simulink model "BSP_v2"  (R2024b)
settings: Solver=VariableStepAuto  StartTime=0.0  StopTime=10.0  RelTol=1e-3
settings Model: Creator=satyendra  LastModifiedBy=satyendra

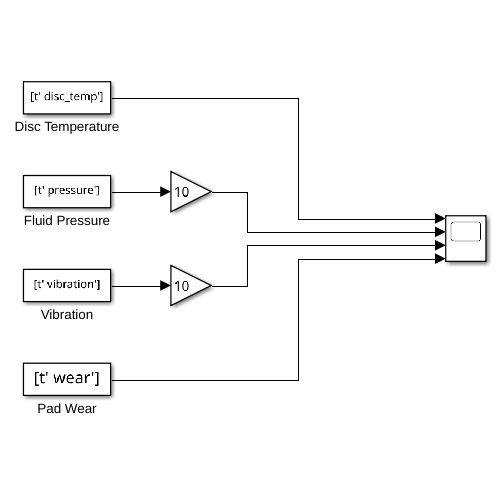
[thumbnail: Simulink's stored preview of the top-level diagram]
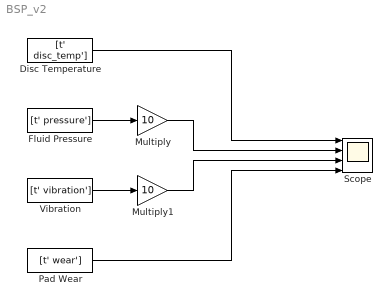
== system BSP_v2 ==
  Disc Temperature : FromWorkspace  VariableName=[t' disc_temp']
  Fluid Pressure : FromWorkspace  VariableName=[t' pressure']
  Multiply : Gain  Gain=10
  Multiply1 : Gain  Gain=10
  Pad Wear : FromWorkspace  VariableName=[t' wear']
  Scope : Scope  NumInputPorts=4
  Vibration : FromWorkspace  VariableName=[t' vibration']
  wires:
  Disc Temperature/1 -> Scope/1
  Fluid Pressure/1 -> Multiply/1
  Vibration/1 -> Multiply1/1
  Pad Wear/1 -> Scope/4
  Multiply1/1 -> Scope/3
  Multiply/1 -> Scope/2
